simulink model "DiplomaSimulink"  (R2017b)
settings: Solver=ode1  StartTime=0.0  StopTime=20  FixedStep=0.0001  RelTol=1e-3
model workspace (MAT data in the model file):
  DiplomaSimulink_sdosession = sldodialogs.data.SessionData
  DiplomaSimulink_sdosession.Version = '3.0'
  DiplomaSimulink_sdosession.Data.ModelName = 'DiplomaSimulink'
  DiplomaSimulink_sdosession.Data.ToolType = 'ResponseOptimization'
  DiplomaSimulink_sdosession.Data.GUIOptions.NoPromptClose = 0
  DiplomaSimulink_sdosession.Data.Workspace.LocalWorkspace.DesignVars(1) = param.Continuous
  DiplomaSimulink_sdosession.Data.Workspace.LocalWorkspace.DesignVars(1).Size_ = [1 1]
  DiplomaSimulink_sdosession.Data.Workspace.LocalWorkspace.DesignVars(1).Value_ = 1
  DiplomaSimulink_sdosession.Data.Workspace.LocalWorkspace.DesignVars(1).pID = paramid.Variable
  DiplomaSimulink_sdosession.Data.Workspace.LocalWorkspace.DesignVars(1).pID.Name = 'KdPitch'
  DiplomaSimulink_sdosession.Data.Workspace.LocalWorkspace.DesignVars(2) = param.Continuous
  DiplomaSimulink_sdosession.Data.Workspace.LocalWorkspace.DesignVars(2).Size_ = [1 1]
  DiplomaSimulink_sdosession.Data.Workspace.LocalWorkspace.DesignVars(2).Value_ = 1
  DiplomaSimulink_sdosession.Data.Workspace.LocalWorkspace.DesignVars(2).pID = paramid.Variable
  DiplomaSimulink_sdosession.Data.Workspace.LocalWorkspace.DesignVars(2).pID.Name = 'KdRoll'
  DiplomaSimulink_sdosession.Data.Workspace.LocalWorkspace.DesignVars(3) = param.Continuous
  DiplomaSimulink_sdosession.Data.Workspace.LocalWorkspace.DesignVars(3).Size_ = [1 1]
  DiplomaSimulink_sdosession.Data.Workspace.LocalWorkspace.DesignVars(3).Value_ = 1
  DiplomaSimulink_sdosession.Data.Workspace.LocalWorkspace.DesignVars(3).pID = paramid.Variable
  DiplomaSimulink_sdosession.Data.Workspace.LocalWorkspace.DesignVars(3).pID.Name = 'KdYaw'
  DiplomaSimulink_sdosession.Data.Workspace.LocalWorkspace.DesignVars(4) = param.Continuous
  DiplomaSimulink_sdosession.Data.Workspace.LocalWorkspace.DesignVars(4).Size_ = [1 1]
  DiplomaSimulink_sdosession.Data.Workspace.LocalWorkspace.DesignVars(4).Value_ = 1
  DiplomaSimulink_sdosession.Data.Workspace.LocalWorkspace.DesignVars(4).pID = paramid.Variable
  DiplomaSimulink_sdosession.Data.Workspace.LocalWorkspace.DesignVars(4).pID.Name = 'KiPitch'
  DiplomaSimulink_sdosession.Data.Workspace.LocalWorkspace.DesignVars(5) = param.Continuous
  DiplomaSimulink_sdosession.Data.Workspace.LocalWorkspace.DesignVars(5).Size_ = [1 1]
  DiplomaSimulink_sdosession.Data.Workspace.LocalWorkspace.DesignVars(5).Value_ = 1
  DiplomaSimulink_sdosession.Data.Workspace.LocalWorkspace.DesignVars(5).pID = paramid.Variable
  DiplomaSimulink_sdosession.Data.Workspace.LocalWorkspace.DesignVars(5).pID.Name = 'KiRoll'
  DiplomaSimulink_sdosession.Data.Workspace.LocalWorkspace.DesignVars(6) = param.Continuous
  DiplomaSimulink_sdosession.Data.Workspace.LocalWorkspace.DesignVars(6).Size_ = [1 1]
  DiplomaSimulink_sdosession.Data.Workspace.LocalWorkspace.DesignVars(6).Value_ = 1
  DiplomaSimulink_sdosession.Data.Workspace.LocalWorkspace.DesignVars(6).pID = paramid.Variable
  DiplomaSimulink_sdosession.Data.Workspace.LocalWorkspace.DesignVars(6).pID.Name = 'KiYaw'
  DiplomaSimulink_sdosession.Data.Workspace.LocalWorkspace.DesignVars(7) = param.Continuous
  DiplomaSimulink_sdosession.Data.Workspace.LocalWorkspace.DesignVars(7).Size_ = [1 1]
  DiplomaSimulink_sdosession.Data.Workspace.LocalWorkspace.DesignVars(7).Value_ = 1
  DiplomaSimulink_sdosession.Data.Workspace.LocalWorkspace.DesignVars(7).pID = paramid.Variable
  DiplomaSimulink_sdosession.Data.Workspace.LocalWorkspace.DesignVars(7).pID.Name = 'KpPitch'
  DiplomaSimulink_sdosession.Data.Workspace.LocalWorkspace.DesignVars(8) = param.Continuous
  DiplomaSimulink_sdosession.Data.Workspace.LocalWorkspace.DesignVars(8).Size_ = [1 1]
  DiplomaSimulink_sdosession.Data.Workspace.LocalWorkspace.DesignVars(8).Value_ = 1
  DiplomaSimulink_sdosession.Data.Workspace.LocalWorkspace.DesignVars(8).pID = paramid.Variable
  DiplomaSimulink_sdosession.Data.Workspace.LocalWorkspace.DesignVars(8).pID.Name = 'KpRoll'
  DiplomaSimulink_sdosession.Data.Workspace.LocalWorkspace.DesignVars(9) = param.Continuous
  DiplomaSimulink_sdosession.Data.Workspace.LocalWorkspace.DesignVars(9).Size_ = [1 1]
  DiplomaSimulink_sdosession.Data.Workspace.LocalWorkspace.DesignVars(9).Value_ = 1
  DiplomaSimulink_sdosession.Data.Workspace.LocalWorkspace.DesignVars(9).pID = paramid.Variable
  DiplomaSimulink_sdosession.Data.Workspace.LocalWorkspace.DesignVars(9).pID.Name = 'KpYaw'
  DiplomaSimulink_sdosession.Data.Workspace.LocalWorkspace.Pitch = Simulink.SimulationData.Signal
  DiplomaSimulink_sdosession.Data.Workspace.LocalWorkspace.Pitch.PortType = 'outport'
  DiplomaSimulink_sdosession.Data.Workspace.LocalWorkspace.Pitch.PortIndex = 2
  DiplomaSimulink_sdosession.Data.Workspace.LocalWorkspace.Pitch.Version = 1
  DiplomaSimulink_sdosession.Data.Workspace.LocalWorkspace.Pitch.BlockPath = Simulink.SimulationData.BlockPath
  DiplomaSimulink_sdosession.Data.Workspace.LocalWorkspace.Pitch.BlockPath.path = {'DiplomaSimulink/QuadCopterModel'}
  DiplomaSimulink_sdosession.Data.Workspace.LocalWorkspace.Pitch.Name = 'Pitch'
  DiplomaSimulink_sdosession.Data.Workspace.LocalWorkspace.PitchStepResponse = sdo.requirements.StepResponseEnvelope
  DiplomaSimulink_sdosession.Data.Workspace.LocalWorkspace.PitchStepResponse.sdo.requirements.Requirement.Data_ : srorequirement.steprespdata (value not decoded)
  DiplomaSimulink_sdosession.Data.Workspace.LocalWorkspace.PitchStepResponse.sdo.requirements.Requirement.Check_ = sdo.requirements.PiecewiseLinearCheck
  DiplomaSimulink_sdosession.Data.Workspace.LocalWorkspace.PitchStepResponse.sdo.requirements.Requirement.Check_.Orientation = 'horizontal'
  DiplomaSimulink_sdosession.Data.Workspace.LocalWorkspace.PitchStepResponse.sdo.requirements.Requirement.Check_.XScale = 'linear'
  DiplomaSimulink_sdosession.Data.Workspace.LocalWorkspace.Roll = Simulink.SimulationData.Signal
  DiplomaSimulink_sdosession.Data.Workspace.LocalWorkspace.Roll.PortType = 'outport'
  DiplomaSimulink_sdosession.Data.Workspace.LocalWorkspace.Roll.Version = 1
  DiplomaSimulink_sdosession.Data.Workspace.LocalWorkspace.Roll.BlockPath = Simulink.SimulationData.BlockPath
  DiplomaSimulink_sdosession.Data.Workspace.LocalWorkspace.Roll.BlockPath.path = {'DiplomaSimulink/QuadCopterModel'}
  DiplomaSimulink_sdosession.Data.Workspace.LocalWorkspace.Roll.Name = 'Roll'
  DiplomaSimulink_sdosession.Data.Workspace.LocalWorkspace.RollStepResponse = sdo.requirements.StepResponseEnvelope
  DiplomaSimulink_sdosession.Data.Workspace.LocalWorkspace.RollStepResponse.sdo.requirements.Requirement.Data_ : srorequirement.steprespdata (value not decoded)
  DiplomaSimulink_sdosession.Data.Workspace.LocalWorkspace.RollStepResponse.sdo.requirements.Requirement.Check_ = sdo.requirements.PiecewiseLinearCheck
  DiplomaSimulink_sdosession.Data.Workspace.LocalWorkspace.RollStepResponse.sdo.requirements.Requirement.Check_.Orientation = 'horizontal'
  DiplomaSimulink_sdosession.Data.Workspace.LocalWorkspace.RollStepResponse.sdo.requirements.Requirement.Check_.XScale = 'linear'
  DiplomaSimulink_sdosession.Data.Workspace.LocalWorkspace.Yaw = Simulink.SimulationData.Signal
  DiplomaSimulink_sdosession.Data.Workspace.LocalWorkspace.Yaw.PortType = 'outport'
  DiplomaSimulink_sdosession.Data.Workspace.LocalWorkspace.Yaw.PortIndex = 3
  DiplomaSimulink_sdosession.Data.Workspace.LocalWorkspace.Yaw.Version = 1
  DiplomaSimulink_sdosession.Data.Workspace.LocalWorkspace.Yaw.BlockPath = Simulink.SimulationData.BlockPath
  DiplomaSimulink_sdosession.Data.Workspace.LocalWorkspace.Yaw.BlockPath.path = {'DiplomaSimulink/QuadCopterModel'}
  DiplomaSimulink_sdosession.Data.Workspace.LocalWorkspace.Yaw.Name = 'Yaw'
  DiplomaSimulink_sdosession.Data.Workspace.LocalWorkspace.YawStepResponse = sdo.requirements.StepResponseEnvelope
  DiplomaSimulink_sdosession.Data.Workspace.LocalWorkspace.YawStepResponse.sdo.requirements.Requirement.Data_ : srorequirement.steprespdata (value not decoded)
  DiplomaSimulink_sdosession.Data.Workspace.LocalWorkspace.YawStepResponse.sdo.requirements.Requirement.Check_ = sdo.requirements.PiecewiseLinearCheck
  DiplomaSimulink_sdosession.Data.Workspace.LocalWorkspace.YawStepResponse.sdo.requirements.Requirement.Check_.Orientation = 'horizontal'
  DiplomaSimulink_sdosession.Data.Workspace.LocalWorkspace.YawStepResponse.sdo.requirements.Requirement.Check_.XScale = 'linear'
  DiplomaSimulink_sdosession.Data.Workspace.HiddenWorkspace = []
  DiplomaSimulink_sdosession.Data.ToolData.PlotManager.Plots(1).Class = 'sldoplots.IterPlot'
  DiplomaSimulink_sdosession.Data.ToolData.PlotManager.Plots(1).Sources = {'DesignVars'}
  DiplomaSimulink_sdosession.Data.ToolData.PlotManager.Plots(2).Class = 'sldoplots.TimePlot'
  DiplomaSimulink_sdosession.Data.ToolData.PlotManager.Plots(2).Sources = {'Yaw'}
  DiplomaSimulink_sdosession.Data.ToolData.PlotManager.Plots(3).Class = 'sldoplots.TimePlot'
  DiplomaSimulink_sdosession.Data.ToolData.PlotManager.Plots(3).Sources = {'Pitch'}
  DiplomaSimulink_sdosession.Data.ToolData.PlotManager.Plots(4).Class = 'sldoplots.TimePlot'
  DiplomaSimulink_sdosession.Data.ToolData.PlotManager.Plots(4).Sources = {'Roll'}
  DiplomaSimulink_sdosession.Data.ToolData.DialogManager = []
  DiplomaSimulink_sdosession.Data.ToolData.ResponseOptimization.Options = sdo.OptimizeOptions
  DiplomaSimulink_sdosession.Data.ToolData.ResponseOptimization.Options.OptimizedModel = 'DiplomaSimulink'
  DiplomaSimulink_sdosession.Data.ToolData.ResponseOptimization.Options.Version = 2
  DiplomaSimulink_sdosession.Data.ToolData.ResponseOptimization.GUIOptions.ModelTimeOut = Inf
  DiplomaSimulink_sdosession.Data.ToolData.ResponseOptimization.GUIOptions.ShowProgress = 1
  DiplomaSimulink_sdosession.Data.ToolData.ResponseOptimization.GUIOptions.ShowParamTrajectory = 1
  DiplomaSimulink_sdosession.Data.ToolData.ResponseOptimization.GUIOptions.UpdatePlots = 1
  DiplomaSimulink_sdosession.Data.ToolData.ResponseOptimization.GUIOptions.UpdateModel = 1
  DiplomaSimulink_sdosession.Data.ToolData.ResponseOptimization.GUIOptions.UpdateDesign = 'overwrite'
  DiplomaSimulink_sdosession.Data.ToolData.ResponseOptimization.GUIOptions.SaveReport = 0
  DiplomaSimulink_sdosession.Data.ToolData.ResponseOptimization.GUIOptions.SaveRequirementValue = 1
  DiplomaSimulink_sdosession.Data.ToolData.ResponseOptimization.LinOptions = linearize.LinearizeOptions
  DiplomaSimulink_sdosession.Data.ToolData.ResponseOptimization.LocalRequirements(1).Requirement = 'YawStepResponse'
  DiplomaSimulink_sdosession.Data.ToolData.ResponseOptimization.LocalRequirements(1).Source = {'Yaw'}
  DiplomaSimulink_sdosession.Data.ToolData.ResponseOptimization.LocalRequirements(1).Selected = 1
  DiplomaSimulink_sdosession.Data.ToolData.ResponseOptimization.LocalRequirements(2).Requirement = 'PitchStepResponse'
  DiplomaSimulink_sdosession.Data.ToolData.ResponseOptimization.LocalRequirements(2).Source = {'Pitch'}
  DiplomaSimulink_sdosession.Data.ToolData.ResponseOptimization.LocalRequirements(2).Selected = 1
  DiplomaSimulink_sdosession.Data.ToolData.ResponseOptimization.LocalRequirements(3).Requirement = 'RollStepResponse'
  DiplomaSimulink_sdosession.Data.ToolData.ResponseOptimization.LocalRequirements(3).Source = {'Roll'}
  DiplomaSimulink_sdosession.Data.ToolData.ResponseOptimization.LocalRequirements(3).Selected = 1
  DiplomaSimulink_sdosession.Data.ToolData.ResponseOptimization.BlockRequirements = struct([])
  DiplomaSimulink_sdosession.Data.ToolData.ResponseOptimization.LocalExperiments = struct([])
  DiplomaSimulink_sdosession.Data.ToolData.ResponseOptimization.Cost.Type = 'SSE'
  DiplomaSimulink_sdosession.Data.ToolData.ResponseOptimization.Cost.Robust = 'off'
  DiplomaSimulink_sdosession.Data.ToolData.ResponseOptimization.DesignVariables = 'DesignVars'
  DiplomaSimulink_sdosession.Data.ToolData.ResponseOptimization.UncertainVariables = ''
  DiplomaSimulink_sdosession.Data.ToolData.ResponseOptimization.DataToPlot = 'Roll'
undefined symbols (not defined in the file or in its folder): KdPitch, KdRoll, KdYaw, KiPitch, KiRoll, KiYaw, KpPitch, KpRoll, KpYaw
libraries: simulink x3
settings Model: Creator=willfordworks  LastModifiedBy=WillfordRockwell
settings CodeAppCC: StateflowObjectComments=on

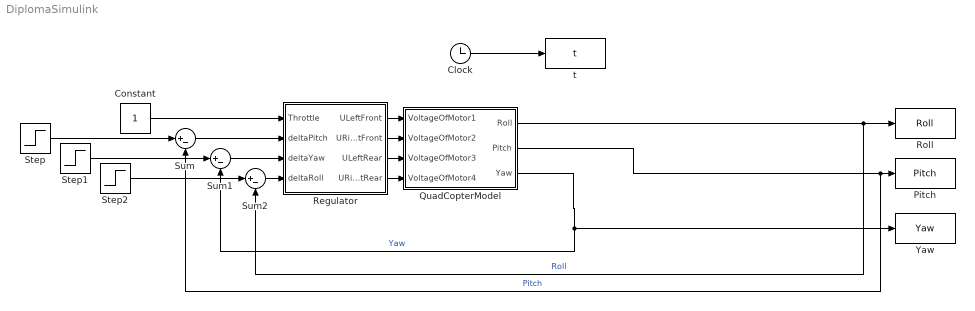
== system DiplomaSimulink ==
  Clock : Clock
  Constant : Constant
  Pitch : ToWorkspace  VariableName=Pitch  SampleTime=-1
  QuadCopterModel : Subsystem
  Regulator : Subsystem
  Roll : ToWorkspace  VariableName=Roll  SampleTime=-1
  Step : Step  SampleTime=0
  Step1 : Step  Time=2  SampleTime=0
  Step2 : Step  Time=3  SampleTime=0
  Sum : Sum  Inputs=|+-
  Sum1 : Sum  Inputs=|+-
  Sum2 : Sum  Inputs=|+-
  Yaw : ToWorkspace  VariableName=Yaw  SampleTime=-1
  t : ToWorkspace  VariableName=t  SampleTime=-1
  wires:
  QuadCopterModel/1(Roll) -> Sum2/2, Roll/1  "Roll"
  QuadCopterModel/2(Pitch) -> Sum/2, Pitch/1  "Pitch"
  QuadCopterModel/3(Yaw) -> Sum1/2, Yaw/1  "Yaw"
  Clock/1 -> t/1
  Regulator/1(ULeftFront) -> QuadCopterModel/1(VoltageOfMotor1)
  Regulator/2(URightFront) -> QuadCopterModel/2(VoltageOfMotor2)
  Regulator/3(ULeftRear) -> QuadCopterModel/3(VoltageOfMotor3)
  Regulator/4(URightRear) -> QuadCopterModel/4(VoltageOfMotor4)
  Constant/1 -> Regulator/1(Throttle)
  Sum/1 -> Regulator/2(deltaPitch)
  Sum1/1 -> Regulator/3(deltaYaw)
  Sum2/1 -> Regulator/4(deltaRoll)
  Step/1 -> Sum/1
  Step1/1 -> Sum1/1
  Step2/1 -> Sum2/1

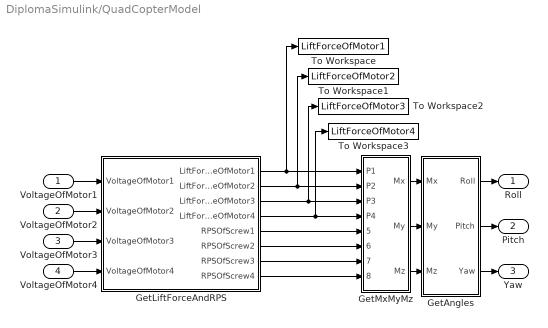
== system DiplomaSimulink/QuadCopterModel ==
  VoltageOfMotor1 : Inport
  VoltageOfMotor2 : Inport  Port=2
  VoltageOfMotor3 : Inport  Port=3
  VoltageOfMotor4 : Inport  Port=4
  GetAngles : Subsystem
  GetLiftForceAndRPS : Subsystem
  GetMxMyMz : Subsystem
  To Workspace : ToWorkspace  VariableName=LiftForceOfMotor1  SampleTime=-1
  To Workspace1 : ToWorkspace  VariableName=LiftForceOfMotor2  SampleTime=-1
  To Workspace2 : ToWorkspace  VariableName=LiftForceOfMotor3  SampleTime=-1
  To Workspace3 : ToWorkspace  VariableName=LiftForceOfMotor4  SampleTime=-1
  Roll : Outport
  Pitch : Outport  Port=2
  Yaw : Outport  Port=3
  wires:
  GetLiftForceAndRPS/1(LiftForceOfMotor1) -> To Workspace/1, GetMxMyMz/1(P1)
  GetLiftForceAndRPS/2(LiftForceOfMotor2) -> To Workspace1/1, GetMxMyMz/2(P2)
  GetLiftForceAndRPS/3(LiftForceOfMotor3) -> To Workspace2/1, GetMxMyMz/3(P3)
  GetLiftForceAndRPS/6(RPSOfScrew2) -> GetMxMyMz/6(RPS2)
  GetLiftForceAndRPS/7(RPSOfScrew3) -> GetMxMyMz/7(RPS3)
  GetLiftForceAndRPS/4(LiftForceOfMotor4) -> To Workspace3/1, GetMxMyMz/4(P4)
  GetLiftForceAndRPS/8(RPSOfScrew4) -> GetMxMyMz/8(RPS4)
  GetLiftForceAndRPS/5(RPSOfScrew1) -> GetMxMyMz/5(RPS1)
  GetAngles/3(Yaw) -> Yaw/1
  GetMxMyMz/2(My) -> GetAngles/2(My)
  GetMxMyMz/1(Mx) -> GetAngles/1(Mx)
  VoltageOfMotor4/1 -> GetLiftForceAndRPS/4(VoltageOfMotor4)
  VoltageOfMotor2/1 -> GetLiftForceAndRPS/2(VoltageOfMotor2)
  GetAngles/2(Pitch) -> Pitch/1
  GetAngles/1(Roll) -> Roll/1
  VoltageOfMotor1/1 -> GetLiftForceAndRPS/1(VoltageOfMotor1)
  GetMxMyMz/3(Mz) -> GetAngles/3(Mz)
  VoltageOfMotor3/1 -> GetLiftForceAndRPS/3(VoltageOfMotor3)

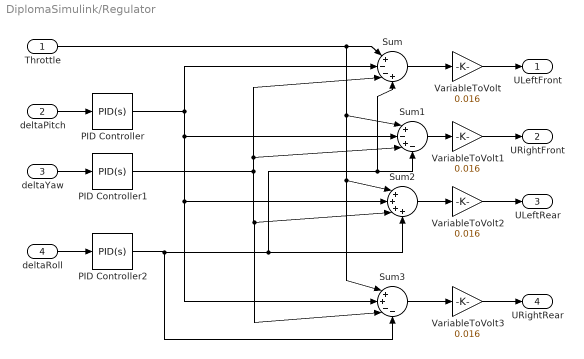
== system DiplomaSimulink/Regulator ==
  Throttle : Inport
  deltaPitch : Inport  Port=2
  deltaYaw : Inport  Port=3
  deltaRoll : Inport  Port=4
  PID Controller : simulink/Continuous/PID Controller  Controller=PID  TimeDomain=Continuous-time  SampleTime=-1  IntegratorMethod=Forward Euler  FilterMethod=Forward Euler  Form=Parallel  UseFilter=on  ControllerParametersSource=internal  P=KpPitch  I=KiPitch  D=KdPitch  N=100  InitialConditionSource=internal  InitialConditionForIntegrator=0  InitialConditionForFilter=0  ExternalReset=none  LimitOutput=off  UpperSaturationLimit=inf  LowerSaturationLimit=-inf  LinearizeAsGain=on  AntiWindupMode=none  Kb=1  TrackingMode=off  Kt=1  PParamMin=[]  PParamMax=[]  IParamMin=[]  IParamMax=[]  DParamMin=[]  DParamMax=[]  NParamMin=[]  NParamMax=[]  KbParamMin=[]  KbParamMax=[]  KtParamMin=[]  KtParamMax=[]  POutMin=[]  POutMax=[]  IOutMin=[]  IOutMax=[]  DOutMin=[]  DOutMax=[]  NOutMin=[]  NOutMax=[]  KbOutMin=[]  KbOutMax=[]  KtOutMin=[]  KtOutMax=[]  IntegratorOutMin=[]  IntegratorOutMax=[]  FilterOutMin=[]  FilterOutMax=[]  SumOutMin=[]  SumOutMax=[]  SumI1OutMin=[]  SumI1OutMax=[]  SumI2OutMin=[]  SumI2OutMax=[]  SumI3OutMin=[]  SumI3OutMax=[]  SumDOutMin=[]  SumDOutMax=[]  SaturationOutMin=[]  SaturationOutMax=[]  IntegratorContinuousStateAttributes=''  IntegratorStateMustResolveToSignalObject=off  IntegratorRTWStateStorageClass=Auto  FilterContinuousStateAttributes=''  FilterStateMustResolveToSignalObject=off  FilterRTWStateStorageClass=Auto  DifferentiatorICPrevScaledInput=0  DifferentiatorOutMin=[]  DifferentiatorOutMax=[]  InitialConditionSetting=State (most efficient)  FilterDiffOutCoefMin=[]  FilterDiffOutCoefMax=[]  SumDenOutMin=[]  SumDenOutMax=[]  SumNumOutMin=[]  SumNumOutMax=[]  ReciprocalOutMin=[]  ReciprocalOutMax=[]  DivideOutMin=[]  DivideOutMax=[]  TunerSelectOption=Transfer Function Based (PID Tuner App)
  PID Controller1 : simulink/Continuous/PID Controller  Controller=PID  TimeDomain=Continuous-time  SampleTime=-1  IntegratorMethod=Forward Euler  FilterMethod=Forward Euler  Form=Parallel  UseFilter=on  ControllerParametersSource=internal  P=KpYaw  I=KiYaw  D=KdYaw  N=100  InitialConditionSource=internal  InitialConditionForIntegrator=0  InitialConditionForFilter=0  ExternalReset=none  LimitOutput=off  UpperSaturationLimit=inf  LowerSaturationLimit=-inf  LinearizeAsGain=on  AntiWindupMode=none  Kb=1  TrackingMode=off  Kt=1  PParamMin=[]  PParamMax=[]  IParamMin=[]  IParamMax=[]  DParamMin=[]  DParamMax=[]  NParamMin=[]  NParamMax=[]  KbParamMin=[]  KbParamMax=[]  KtParamMin=[]  KtParamMax=[]  POutMin=[]  POutMax=[]  IOutMin=[]  IOutMax=[]  DOutMin=[]  DOutMax=[]  NOutMin=[]  NOutMax=[]  KbOutMin=[]  KbOutMax=[]  KtOutMin=[]  KtOutMax=[]  IntegratorOutMin=[]  IntegratorOutMax=[]  FilterOutMin=[]  FilterOutMax=[]  SumOutMin=[]  SumOutMax=[]  SumI1OutMin=[]  SumI1OutMax=[]  SumI2OutMin=[]  SumI2OutMax=[]  SumI3OutMin=[]  SumI3OutMax=[]  SumDOutMin=[]  SumDOutMax=[]  SaturationOutMin=[]  SaturationOutMax=[]  IntegratorContinuousStateAttributes=''  IntegratorStateMustResolveToSignalObject=off  IntegratorRTWStateStorageClass=Auto  FilterContinuousStateAttributes=''  FilterStateMustResolveToSignalObject=off  FilterRTWStateStorageClass=Auto  DifferentiatorICPrevScaledInput=0  DifferentiatorOutMin=[]  DifferentiatorOutMax=[]  InitialConditionSetting=State (most efficient)  FilterDiffOutCoefMin=[]  FilterDiffOutCoefMax=[]  SumDenOutMin=[]  SumDenOutMax=[]  SumNumOutMin=[]  SumNumOutMax=[]  ReciprocalOutMin=[]  ReciprocalOutMax=[]  DivideOutMin=[]  DivideOutMax=[]  TunerSelectOption=Transfer Function Based (PID Tuner App)
  PID Controller2 : simulink/Continuous/PID Controller  Controller=PID  TimeDomain=Continuous-time  SampleTime=-1  IntegratorMethod=Forward Euler  FilterMethod=Forward Euler  Form=Parallel  UseFilter=on  ControllerParametersSource=internal  P=KpRoll  I=KiRoll  D=KdRoll  N=100  InitialConditionSource=internal  InitialConditionForIntegrator=0  InitialConditionForFilter=0  ExternalReset=none  LimitOutput=off  UpperSaturationLimit=inf  LowerSaturationLimit=-inf  LinearizeAsGain=on  AntiWindupMode=none  Kb=1  TrackingMode=off  Kt=1  PParamMin=[]  PParamMax=[]  IParamMin=[]  IParamMax=[]  DParamMin=[]  DParamMax=[]  NParamMin=[]  NParamMax=[]  KbParamMin=[]  KbParamMax=[]  KtParamMin=[]  KtParamMax=[]  POutMin=[]  POutMax=[]  IOutMin=[]  IOutMax=[]  DOutMin=[]  DOutMax=[]  NOutMin=[]  NOutMax=[]  KbOutMin=[]  KbOutMax=[]  KtOutMin=[]  KtOutMax=[]  IntegratorOutMin=[]  IntegratorOutMax=[]  FilterOutMin=[]  FilterOutMax=[]  SumOutMin=[]  SumOutMax=[]  SumI1OutMin=[]  SumI1OutMax=[]  SumI2OutMin=[]  SumI2OutMax=[]  SumI3OutMin=[]  SumI3OutMax=[]  SumDOutMin=[]  SumDOutMax=[]  SaturationOutMin=[]  SaturationOutMax=[]  IntegratorContinuousStateAttributes=''  IntegratorStateMustResolveToSignalObject=off  IntegratorRTWStateStorageClass=Auto  FilterContinuousStateAttributes=''  FilterStateMustResolveToSignalObject=off  FilterRTWStateStorageClass=Auto  DifferentiatorICPrevScaledInput=0  DifferentiatorOutMin=[]  DifferentiatorOutMax=[]  InitialConditionSetting=State (most efficient)  FilterDiffOutCoefMin=[]  FilterDiffOutCoefMax=[]  SumDenOutMin=[]  SumDenOutMax=[]  SumNumOutMin=[]  SumNumOutMax=[]  ReciprocalOutMin=[]  ReciprocalOutMax=[]  DivideOutMin=[]  DivideOutMax=[]  TunerSelectOption=Transfer Function Based (PID Tuner App)
  Sum : Sum  Inputs=|+--+
  Sum1 : Sum  Inputs=|+-+-
  Sum2 : Sum  Inputs=|++++
  Sum3 : Sum  Inputs=|++--
  VariableToVolt{,1..3} (4 alike) : Gain  Gain=0.016
  ULeftFront : Outport
  URightFront : Outport  Port=2
  ULeftRear : Outport  Port=3
  URightRear : Outport  Port=4
  wires:
  deltaRoll/1 -> PID Controller2/1
  deltaPitch/1 -> PID Controller/1
  Throttle/1 -> Sum1/1, Sum3/1, Sum2/1, Sum/1
  deltaYaw/1 -> PID Controller1/1
  Sum/1 -> VariableToVolt/1
  Sum1/1 -> VariableToVolt1/1
  Sum2/1 -> VariableToVolt2/1
  Sum3/1 -> VariableToVolt3/1
  VariableToVolt/1 -> ULeftFront/1
  VariableToVolt1/1 -> URightFront/1
  VariableToVolt2/1 -> ULeftRear/1
  VariableToVolt3/1 -> URightRear/1
  PID Controller/1 -> Sum1/2, Sum3/2, Sum2/2, Sum/2
  PID Controller1/1 -> Sum3/3, Sum2/3, Sum1/3, Sum/3
  PID Controller2/1 -> Sum1/4, Sum/4, Sum2/4, Sum3/4

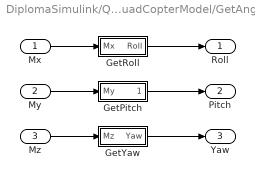
== system DiplomaSimulink/QuadCopterModel/GetAngles ==
  Mx : Inport
  My : Inport  Port=2
  Mz : Inport  Port=3
  GetPitch : Subsystem
  GetRoll : Subsystem
  GetYaw : Subsystem
  Roll : Outport
  Pitch : Outport  Port=2
  Yaw : Outport  Port=3
  wires:
  Mx/1 -> GetRoll/1(Mx)
  My/1 -> GetPitch/1(My)
  Mz/1 -> GetYaw/1(Mz)
  GetYaw/1(Yaw) -> Yaw/1
  GetPitch/1(Pitch) -> Pitch/1
  GetRoll/1(Roll) -> Roll/1

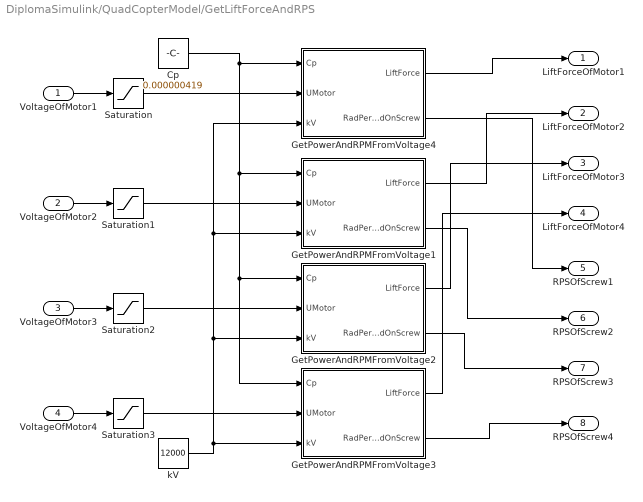
== system DiplomaSimulink/QuadCopterModel/GetLiftForceAndRPS ==
  VoltageOfMotor1 : Inport
  VoltageOfMotor2 : Inport  Port=2
  VoltageOfMotor3 : Inport  Port=3
  VoltageOfMotor4 : Inport  Port=4
  Cp : Constant  Value=0.000000419
  GetPowerAndRPMFromVoltage1 : Subsystem
  GetPowerAndRPMFromVoltage2 : Subsystem
  GetPowerAndRPMFromVoltage3 : Subsystem
  GetPowerAndRPMFromVoltage4 : Subsystem
  Saturation{,1..3} (4 alike) : Saturate  UpperLimit=4.2  LowerLimit=0
  kV : Constant  Value=12000
  LiftForceOfMotor1 : Outport
  LiftForceOfMotor2 : Outport  Port=2
  LiftForceOfMotor3 : Outport  Port=3
  LiftForceOfMotor4 : Outport  Port=4
  RPSOfScrew1 : Outport  Port=5
  RPSOfScrew2 : Outport  Port=6
  RPSOfScrew3 : Outport  Port=7
  RPSOfScrew4 : Outport  Port=8
  wires:
  GetPowerAndRPMFromVoltage3/1(LiftForce) -> LiftForceOfMotor4/1
  GetPowerAndRPMFromVoltage2/1(LiftForce) -> LiftForceOfMotor3/1
  GetPowerAndRPMFromVoltage1/1(LiftForce) -> LiftForceOfMotor2/1
  Cp/1 -> GetPowerAndRPMFromVoltage4/1(Cp), GetPowerAndRPMFromVoltage1/1(Cp), GetPowerAndRPMFromVoltage3/1(Cp), GetPowerAndRPMFromVoltage2/1(Cp)
  GetPowerAndRPMFromVoltage4/1(LiftForce) -> LiftForceOfMotor1/1
  kV/1 -> GetPowerAndRPMFromVoltage3/3(kV), GetPowerAndRPMFromVoltage2/3(kV), GetPowerAndRPMFromVoltage4/3(kV), GetPowerAndRPMFromVoltage1/3(kV)
  GetPowerAndRPMFromVoltage4/2(RadPerSecondOnScrew) -> RPSOfScrew1/1
  GetPowerAndRPMFromVoltage1/2(RadPerSecondOnScrew) -> RPSOfScrew2/1
  GetPowerAndRPMFromVoltage2/2(RadPerSecondOnScrew) -> RPSOfScrew3/1
  GetPowerAndRPMFromVoltage3/2(RadPerSecondOnScrew) -> RPSOfScrew4/1
  VoltageOfMotor2/1 -> Saturation1/1
  Saturation1/1 -> GetPowerAndRPMFromVoltage1/2(UMotor)
  VoltageOfMotor3/1 -> Saturation2/1
  Saturation2/1 -> GetPowerAndRPMFromVoltage2/2(UMotor)
  VoltageOfMotor1/1 -> Saturation/1
  Saturation/1 -> GetPowerAndRPMFromVoltage4/2(UMotor)
  VoltageOfMotor4/1 -> Saturation3/1
  Saturation3/1 -> GetPowerAndRPMFromVoltage3/2(UMotor)

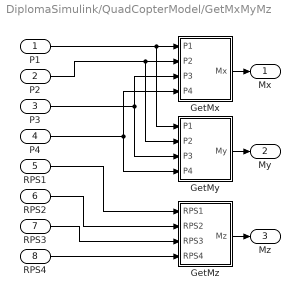
== system DiplomaSimulink/QuadCopterModel/GetMxMyMz ==
  P1 : Inport
  P2 : Inport  Port=2
  P3 : Inport  Port=3
  P4 : Inport  Port=4
  RPS1 : Inport  Port=5
  RPS2 : Inport  Port=6
  RPS3 : Inport  Port=7
  RPS4 : Inport  Port=8
  GetMx : Subsystem
  GetMy : Subsystem
  GetMz : Subsystem
  Mx : Outport
  My : Outport  Port=2
  Mz : Outport  Port=3
  wires:
  GetMy/1(My) -> My/1
  RPS4/1 -> GetMz/4(RPS4)
  GetMz/1(Mz) -> Mz/1
  RPS1/1 -> GetMz/1(RPS1)
  RPS3/1 -> GetMz/3(RPS3)
  GetMx/1(Mx) -> Mx/1
  P1/1 -> GetMx/1(P1), GetMy/1(P1)
  P2/1 -> GetMy/2(P2), GetMx/2(P2)
  P3/1 -> GetMx/3(P3), GetMy/3(P3)
  P4/1 -> GetMx/4(P4), GetMy/4(P4)
  RPS2/1 -> GetMz/2(RPS2)

== system DiplomaSimulink/QuadCopterModel/GetAngles/GetPitch ==
  My : Inport
  Divide : Product  Inputs=*/
  Integrator : Integrator
  Integrator1 : Integrator
  Iy : Constant  Value=0.000247
  Pitch : Outport
  wires:
  My/1 -> Divide/1
  Iy/1 -> Divide/2
  Divide/1 -> Integrator/1
  Integrator/1 -> Integrator1/1
  Integrator1/1 -> Pitch/1

== system DiplomaSimulink/QuadCopterModel/GetAngles/GetRoll ==
  Mx : Inport
  Divide : Product  Inputs=*/
  Integrator : Integrator
  Integrator1 : Integrator
  Ix : Constant  Value=0.000209
  Roll : Outport
  wires:
  Mx/1 -> Divide/1
  Ix/1 -> Divide/2
  Divide/1 -> Integrator/1
  Integrator/1 -> Integrator1/1
  Integrator1/1 -> Roll/1

== system DiplomaSimulink/QuadCopterModel/GetAngles/GetYaw ==
  Mz : Inport
  Divide : Product  Inputs=*/
  Integrator : Integrator
  Integrator1 : Integrator
  Iz : Constant  Value=0.000246
  Yaw : Outport
  wires:
  Mz/1 -> Divide/1
  Iz/1 -> Divide/2
  Divide/1 -> Integrator/1
  Integrator/1 -> Integrator1/1
  Integrator1/1 -> Yaw/1

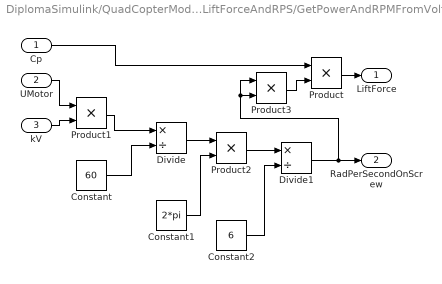
== system DiplomaSimulink/QuadCopterModel/GetLiftForceAndRPS/GetPowerAndRPMFromVoltage1 ==
  Cp : Inport
  UMotor : Inport  Port=2
  kV : Inport  Port=3
  Constant : Constant  Value=60
  Constant1 : Constant  Value=2*pi
  Constant2 : Constant  Value=6
  Divide : Product  Inputs=*/
  Divide1 : Product  Inputs=*/
  Product{,1..3} (4 alike) : Product
  LiftForce : Outport
  RadPerSecondOnScrew : Outport  Port=2
  wires:
  Cp/1 -> Product/1
  Product/1 -> LiftForce/1
  Product1/1 -> Divide/1
  UMotor/1 -> Product1/1
  kV/1 -> Product1/2
  Constant/1 -> Divide/2
  Divide/1 -> Product2/1
  Constant1/1 -> Product2/2
  Product2/1 -> Divide1/1
  Divide1/1 -> Product3/1, Product3/2, RadPerSecondOnScrew/1
  Constant2/1 -> Divide1/2
  Product3/1 -> Product/2

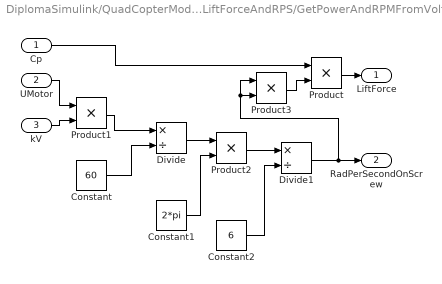
== system DiplomaSimulink/QuadCopterModel/GetLiftForceAndRPS/GetPowerAndRPMFromVoltage2 ==
  Cp : Inport
  UMotor : Inport  Port=2
  kV : Inport  Port=3
  Constant : Constant  Value=60
  Constant1 : Constant  Value=2*pi
  Constant2 : Constant  Value=6
  Divide : Product  Inputs=*/
  Divide1 : Product  Inputs=*/
  Product{,1..3} (4 alike) : Product
  LiftForce : Outport
  RadPerSecondOnScrew : Outport  Port=2
  wires:
  Cp/1 -> Product/1
  Product/1 -> LiftForce/1
  Product1/1 -> Divide/1
  UMotor/1 -> Product1/1
  kV/1 -> Product1/2
  Constant/1 -> Divide/2
  Divide/1 -> Product2/1
  Constant1/1 -> Product2/2
  Product2/1 -> Divide1/1
  Divide1/1 -> Product3/1, Product3/2, RadPerSecondOnScrew/1
  Constant2/1 -> Divide1/2
  Product3/1 -> Product/2

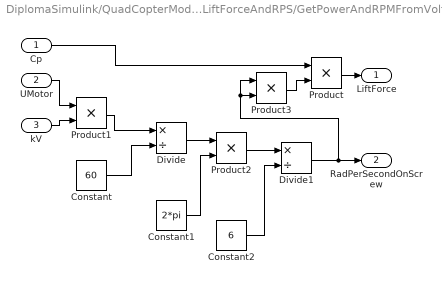
== system DiplomaSimulink/QuadCopterModel/GetLiftForceAndRPS/GetPowerAndRPMFromVoltage3 ==
  Cp : Inport
  UMotor : Inport  Port=2
  kV : Inport  Port=3
  Constant : Constant  Value=60
  Constant1 : Constant  Value=2*pi
  Constant2 : Constant  Value=6
  Divide : Product  Inputs=*/
  Divide1 : Product  Inputs=*/
  Product{,1..3} (4 alike) : Product
  LiftForce : Outport
  RadPerSecondOnScrew : Outport  Port=2
  wires:
  Cp/1 -> Product/1
  Product/1 -> LiftForce/1
  Product1/1 -> Divide/1
  UMotor/1 -> Product1/1
  kV/1 -> Product1/2
  Constant/1 -> Divide/2
  Divide/1 -> Product2/1
  Constant1/1 -> Product2/2
  Product2/1 -> Divide1/1
  Divide1/1 -> Product3/1, Product3/2, RadPerSecondOnScrew/1
  Constant2/1 -> Divide1/2
  Product3/1 -> Product/2

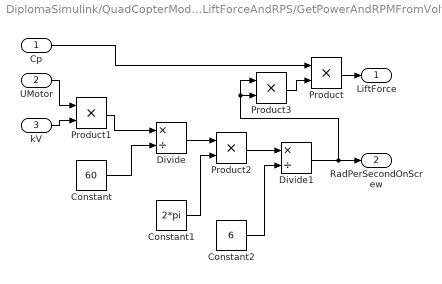
== system DiplomaSimulink/QuadCopterModel/GetLiftForceAndRPS/GetPowerAndRPMFromVoltage4 ==
  Cp : Inport
  UMotor : Inport  Port=2
  kV : Inport  Port=3
  Constant : Constant  Value=60
  Constant1 : Constant  Value=2*pi
  Constant2 : Constant  Value=6
  Divide : Product  Inputs=*/
  Divide1 : Product  Inputs=*/
  Product{,1..3} (4 alike) : Product
  LiftForce : Outport
  RadPerSecondOnScrew : Outport  Port=2
  wires:
  Cp/1 -> Product/1
  Product/1 -> LiftForce/1
  Product1/1 -> Divide/1
  UMotor/1 -> Product1/1
  kV/1 -> Product1/2
  Constant/1 -> Divide/2
  Divide/1 -> Product2/1
  Constant1/1 -> Product2/2
  Product2/1 -> Divide1/1
  Divide1/1 -> Product3/1, Product3/2, RadPerSecondOnScrew/1
  Constant2/1 -> Divide1/2
  Product3/1 -> Product/2

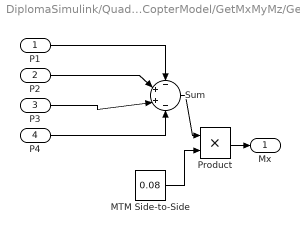
== system DiplomaSimulink/QuadCopterModel/GetMxMyMz/GetMx ==
  P1 : Inport
  P2 : Inport  Port=2
  P3 : Inport  Port=3
  P4 : Inport  Port=4
  MTM Side-to-Side : Constant  Value=0.08
  Product : Product
  Sum : Sum  Inputs=-++-
  Mx : Outport
  wires:
  Sum/1 -> Product/1
  MTM Side-to-Side/1 -> Product/2
  P1/1 -> Sum/1
  P4/1 -> Sum/4
  P2/1 -> Sum/2
  P3/1 -> Sum/3
  Product/1 -> Mx/1

== system DiplomaSimulink/QuadCopterModel/GetMxMyMz/GetMy ==
  P1 : Inport
  P2 : Inport  Port=2
  P3 : Inport  Port=3
  P4 : Inport  Port=4
  MTM Side-to-Side : Constant  Value=0.08
  Product : Product
  Sum : Sum  Inputs=++--
  My : Outport
  wires:
  Sum/1 -> Product/1
  MTM Side-to-Side/1 -> Product/2
  P1/1 -> Sum/1
  P4/1 -> Sum/4
  P2/1 -> Sum/2
  P3/1 -> Sum/3
  Product/1 -> My/1

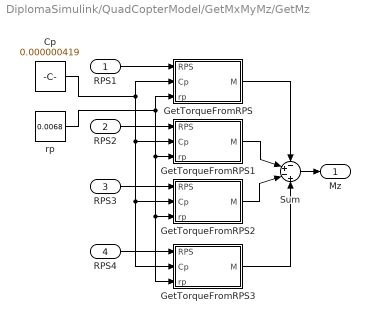
== system DiplomaSimulink/QuadCopterModel/GetMxMyMz/GetMz ==
  RPS1 : Inport
  RPS2 : Inport  Port=2
  RPS3 : Inport  Port=3
  RPS4 : Inport  Port=4
  Cp : Constant  Value=0.000000419
  GetTorqueFromRPS : Subsystem
  GetTorqueFromRPS1 : Subsystem
  GetTorqueFromRPS2 : Subsystem
  GetTorqueFromRPS3 : Subsystem
  Sum : Sum  Inputs=-+-+
  rp : Constant  Value=0.0068
  Mz : Outport
  wires:
  Sum/1 -> Mz/1
  RPS1/1 -> GetTorqueFromRPS/1(RPS)
  GetTorqueFromRPS/1(M) -> Sum/1
  GetTorqueFromRPS1/1(M) -> Sum/2
  RPS2/1 -> GetTorqueFromRPS1/1(RPS)
  GetTorqueFromRPS2/1(M) -> Sum/3
  RPS3/1 -> GetTorqueFromRPS2/1(RPS)
  GetTorqueFromRPS3/1(M) -> Sum/4
  RPS4/1 -> GetTorqueFromRPS3/1(RPS)
  rp/1 -> GetTorqueFromRPS/3(rp), GetTorqueFromRPS3/3(rp), GetTorqueFromRPS2/3(rp), GetTorqueFromRPS1/3(rp)
  Cp/1 -> GetTorqueFromRPS3/2(Cp), GetTorqueFromRPS2/2(Cp), GetTorqueFromRPS1/2(Cp), GetTorqueFromRPS/2(Cp)

== system DiplomaSimulink/QuadCopterModel/GetMxMyMz/GetMz/GetTorqueFromRPS ==
  RPS : Inport
  Cp : Inport  Port=2
  rp : Inport  Port=3
  Product : Product
  Product1 : Product
  Product2 : Product
  M : Outport
  wires:
  RPS/1 -> Product/2, Product/1
  Cp/1 -> Product1/2
  Product/1 -> Product1/1
  Product1/1 -> Product2/1
  rp/1 -> Product2/2
  Product2/1 -> M/1

== system DiplomaSimulink/QuadCopterModel/GetMxMyMz/GetMz/GetTorqueFromRPS1 ==
  RPS : Inport
  Cp : Inport  Port=2
  rp : Inport  Port=3
  Product : Product
  Product1 : Product
  Product2 : Product
  M : Outport
  wires:
  RPS/1 -> Product/2, Product/1
  Cp/1 -> Product1/2
  Product/1 -> Product1/1
  Product1/1 -> Product2/1
  rp/1 -> Product2/2
  Product2/1 -> M/1

== system DiplomaSimulink/QuadCopterModel/GetMxMyMz/GetMz/GetTorqueFromRPS2 ==
  RPS : Inport
  Cp : Inport  Port=2
  rp : Inport  Port=3
  Product : Product
  Product1 : Product
  Product2 : Product
  M : Outport
  wires:
  RPS/1 -> Product/2, Product/1
  Cp/1 -> Product1/2
  Product/1 -> Product1/1
  Product1/1 -> Product2/1
  rp/1 -> Product2/2
  Product2/1 -> M/1

== system DiplomaSimulink/QuadCopterModel/GetMxMyMz/GetMz/GetTorqueFromRPS3 ==
  RPS : Inport
  Cp : Inport  Port=2
  rp : Inport  Port=3
  Product : Product
  Product1 : Product
  Product2 : Product
  M : Outport
  wires:
  RPS/1 -> Product/2, Product/1
  Cp/1 -> Product1/2
  Product/1 -> Product1/1
  Product1/1 -> Product2/1
  rp/1 -> Product2/2
  Product2/1 -> M/1
